simulink model "simu_control_robot_6"  (Simulink 7.9)
settings: Solver=ode3  StartTime=0.0  StopTime=1.2  FixedStep=0.01  RelTol=1e-3
values from neighbouring files (symbols this model uses):
  w = wpg_param.w    [WPG_results.m]    (also in WPG_results_10.m; WPG_results_2.m; WPG_results_3.m; WPG_results_4.m)
  xsx_d = repmat(0,duration_disc,1)    [WPG_results_10.m]    (also in WPG_results_2.m = zmp.A_xcom_spd(1:sum(wpg_param.discretization(1:wpg_param.nb; WPG_results_3.m = zmp.A_xcom_spd(1:sum(wpg_param.discretization(1:wpg_param.nb; WPG_results_4.m = repmat(zmp.A_xcom_spd(1,:)*wpg_param.psa_abcdDSP(1:size(zmp.; WPG_results_5.m = [time xsx_d-xsx_d_init])
  xx_d = repmat(trajectories_zmp.xpcom(1),duration_disc,1)    [WPG_results_10.m]    (also in WPG_results_2.m = trajectories_zmp.xpcom(1:sum(wpg_param.discretization(1:wpg_; WPG_results_3.m = trajectories_zmp.xpcom(1:sum(wpg_param.discretization(1:wpg_; WPG_results_4.m; WPG_results_5.m = [time xx_d-xx_d_init])
  ysx_d = repmat(0,duration_disc,1)    [WPG_results_10.m]    (also in WPG_results_2.m = zmp.A_ycom_spd(1:sum(wpg_param.discretization(1:wpg_param.nb; WPG_results_3.m = zmp.A_ycom_spd(1:sum(wpg_param.discretization(1:wpg_param.nb; WPG_results_4.m = repmat(zmp.A_ycom_spd(1,:)*wpg_param.psa_abcdDSP(end/2+1:end; WPG_results_5.m = [time ysx_d-ysx_d_init])
  yx_d = repmat(0,duration_disc,1)    [WPG_results_10.m]    (also in WPG_results_2.m = trajectories_zmp.ypcom(1:sum(wpg_param.discretization(1:wpg_; WPG_results_3.m = trajectories_zmp.ypcom(1:sum(wpg_param.discretization(1:wpg_; WPG_results_4.m = repmat(trajectories_zmp.ypcom(1),duration_disc,1); WPG_results_5.m = [time yx_d-yx_d_init])
undefined symbols (not defined in the file or in its folder): wpg_param
settings Model: Creator=pajon  LastModifiedBy=pajon

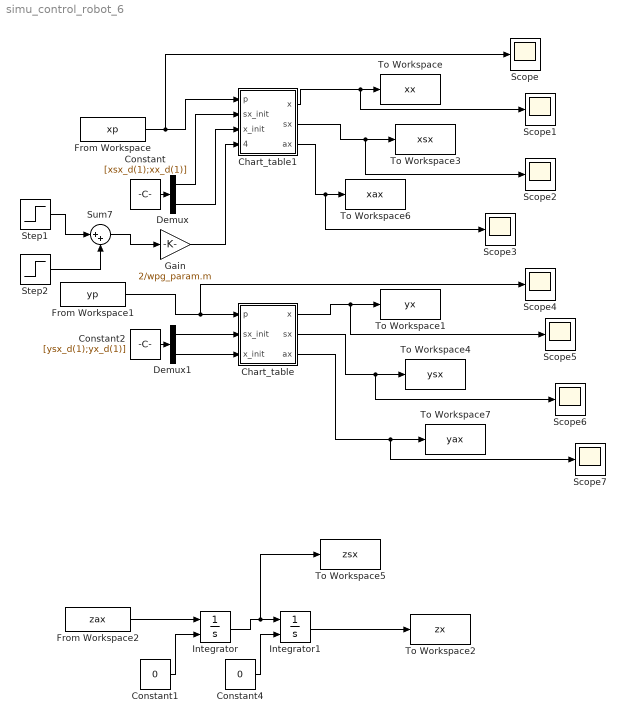
== system simu_control_robot_6 ==
  Chart_table : Subsystem
  Chart_table1 : Subsystem
  Constant : Constant  Value=[xsx_d(1);xx_d(1)]
  Constant1 : Constant  Value=0
  Constant2 : Constant  Value=[ysx_d(1);yx_d(1)]
  Constant4 : Constant  Value=0
  Demux : Demux  Outputs=2
  Demux1 : Demux  Outputs=2
  From Workspace : FromWorkspace  VariableName=xp  SampleTime=0
  From Workspace1 : FromWorkspace  VariableName=yp  SampleTime=0
  From Workspace2 : FromWorkspace  VariableName=zax  SampleTime=0
  Gain : Gain  Gain=2/wpg_param.m
  Integrator : Integrator  InitialConditionSource=external  InitialCondition=xsx_d(1,2)
  Integrator1 : Integrator  InitialConditionSource=external  InitialCondition=xx_d(1,2)
  Scope{,1..7} (8 alike) : Scope
      Scope1 settings: TimeRange=1.2
      Scope2 settings: SaveName=ScopeData2
      Scope3 settings: SaveName=ScopeData3
      Scope4 settings: SaveName=ScopeData4
      Scope5 settings: SaveName=ScopeData5
      Scope6 settings: SaveName=ScopeData6
      Scope7 settings: SaveName=ScopeData7
  Step1 : Step  Time=0.4  After=+2  SampleTime=0
  Step2 : Step  Time=1.5  After=-2  SampleTime=0
  Sum7 : Sum  Inputs=|++
  To Workspace : ToWorkspace  VariableName=xx  SampleTime=-1  SaveFormat=Timeseries
  To Workspace1 : ToWorkspace  VariableName=yx  SampleTime=-1  SaveFormat=Timeseries
  To Workspace2 : ToWorkspace  VariableName=zx  SampleTime=-1  SaveFormat=Timeseries
  To Workspace3 : ToWorkspace  VariableName=xsx  SampleTime=-1  SaveFormat=Timeseries
  To Workspace4 : ToWorkspace  VariableName=ysx  SampleTime=-1  SaveFormat=Timeseries
  To Workspace5 : ToWorkspace  VariableName=zsx  SampleTime=-1  SaveFormat=Timeseries
  To Workspace6 : ToWorkspace  VariableName=xax  SampleTime=-1  SaveFormat=Timeseries
  To Workspace7 : ToWorkspace  VariableName=yax  SampleTime=-1  SaveFormat=Timeseries
  wires:
  Constant2/1 -> Demux1/1
  Constant/1 -> Demux/1
  Integrator/1 -> Integrator1/1, To Workspace5/1
  Constant1/1 -> Integrator/2
  Constant4/1 -> Integrator1/2
  From Workspace2/1 -> Integrator/1
  Integrator1/1 -> To Workspace2/1
  Chart_table1/1(x) -> To Workspace/1, Scope1/1
  Chart_table1/2(sx) -> To Workspace3/1, Scope2/1
  From Workspace/1 -> Chart_table1/1(p), Scope/1
  From Workspace1/1 -> Chart_table/1(p), Scope4/1
  Demux/1 -> Chart_table1/2(sx_init)
  Demux/2 -> Chart_table1/3(x_init)
  Demux1/1 -> Chart_table/2(sx_init)
  Demux1/2 -> Chart_table/3(x_init)
  Chart_table/1(x) -> To Workspace1/1, Scope5/1
  Chart_table/2(sx) -> To Workspace4/1, Scope6/1
  Chart_table1/3(ax) -> To Workspace6/1, Scope3/1
  Chart_table/3(ax) -> To Workspace7/1, Scope7/1
  Step1/1 -> Sum7/1
  Step2/1 -> Sum7/2
  Sum7/1 -> Gain/1
  Gain/1 -> Chart_table1/4(F_perturb)

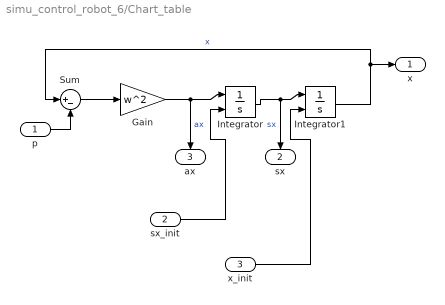
== system simu_control_robot_6/Chart_table ==
  p : Inport
  sx_init : Inport  Port=2
  x_init : Inport  Port=3
  Gain : Gain  Gain=w^2
  Integrator : Integrator  InitialConditionSource=external  InitialCondition=xsx_d(1,2)
  Integrator1 : Integrator  InitialConditionSource=external  InitialCondition=xx_d(1,2)
  Sum : Sum  Inputs=|+-
  x : Outport
  sx : Outport  Port=2
  ax : Outport  Port=3
  wires:
  Integrator/1 -> Integrator1/1, sx/1  "sx"
  Integrator1/1 -> Sum/1, x/1  "x"
  Gain/1 -> Integrator/1, ax/1  "ax"
  Sum/1 -> Gain/1
  p/1 -> Sum/2
  sx_init/1 -> Integrator/2
  x_init/1 -> Integrator1/2

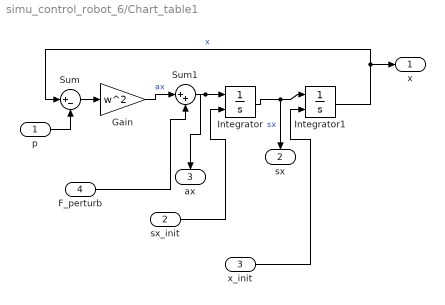
== system simu_control_robot_6/Chart_table1 ==
  p : Inport
  sx_init : Inport  Port=2
  x_init : Inport  Port=3
  F_perturb : Inport  Port=4
  Gain : Gain  Gain=w^2
  Integrator : Integrator  InitialConditionSource=external  InitialCondition=xsx_d(1,2)
  Integrator1 : Integrator  InitialConditionSource=external  InitialCondition=xx_d(1,2)
  Sum : Sum  Inputs=|+-
  Sum1 : Sum  Inputs=|++
  x : Outport
  sx : Outport  Port=2
  ax : Outport  Port=3
  wires:
  Integrator/1 -> Integrator1/1, sx/1  "sx"
  Integrator1/1 -> Sum/1, x/1  "x"
  Sum/1 -> Gain/1
  p/1 -> Sum/2
  sx_init/1 -> Integrator/2
  x_init/1 -> Integrator1/2
  Gain/1 -> Sum1/1  "ax"
  Sum1/1 -> Integrator/1, ax/1
  F_perturb/1 -> Sum1/2
